simulink model "sixythree_level_modified"  (R2020a)
settings: Solver=ode45  StartTime=0.0  StopTime=0.02  RelTol=1e-3  EnableMultiTasking=on
libraries: powerlib x25
settings Model: Creator=harish  LastModifiedBy=sunil
settings DataIOCC: LimitDataPoints=on  SaveFormat=Array  ReturnWorkspaceOutputs=off
settings OptimizationCC: LifeSpan=inf
settings DebuggingCC: SFUnexpectedBacktrackingDiag=warning  SFNoUnconditionalDefaultTransitionDiag=warning  SFExecutionAtInitializationDiag=none  ArithmeticOperatorsInVariantConditions=warning
settings HardwareCC: ProdBitPerPointer=32  ProdBitPerSizeT=32  ProdBitPerPtrDiffT=32  ProdLargestAtomicFloat=None  ProdIntDivRoundTo=Undefined  ProdEndianess=Unspecified  ProdWordSize=32  ProdHWDeviceType=32-bit Generic
settings ModelReferenceCC: PropagateSignalLabelsOutOfModel=off
settings SFSimCC: SimUseLocalCustomCode=off  CustomCodeUndefinedFunction=UseInterfaceOnly
settings RTWCC: RTWUseLocalCustomCode=off
settings CodeAppCC: StateflowObjectComments=on
settings GRTTargetCC: TargetLangStandard=C89/C90 (ANSI)
settings ConfigComp: CovMetricSettings=dw  CovHtmlReporting=on  CovSaveCumulativeToWorkspaceVar=on  CovSaveSingleToWorkspaceVar=on  CovExternalEMLEnable=off
settings SimscapeCC: SimscapeNormalizeSystem=off

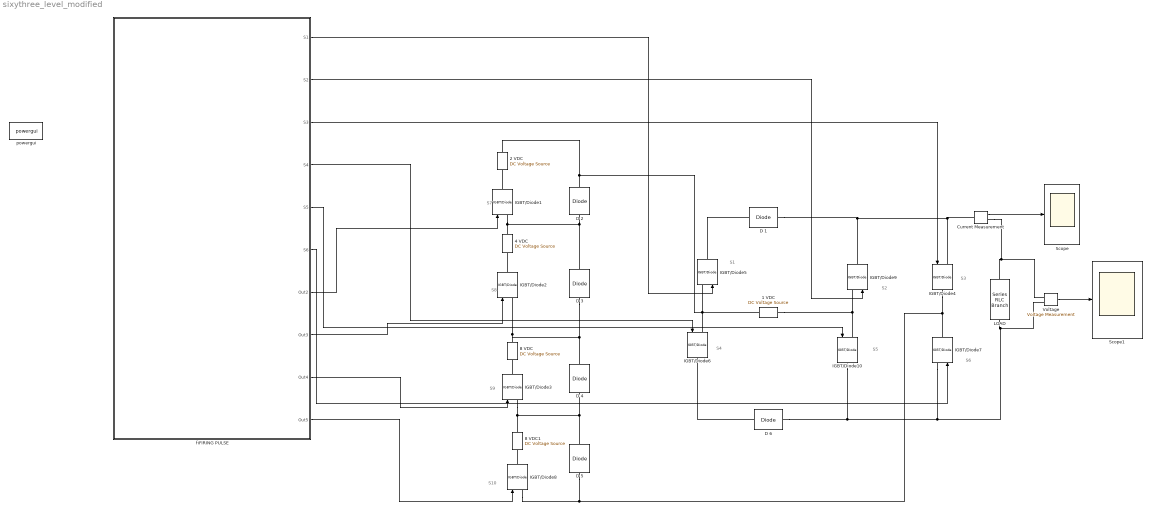
== system sixythree_level_modified ==
  note: S10
  note: S9
  note: S8
  note: S7
  note: S6
  note: S5
  note: S4
  note: S3
  note: S2
  note: S1
   D {1..6} (6 alike) : powerlib/Power Electronics/Diode  Ron=0.001  Lon=0  Vf=0.8  IC=0  UseSnubber=off  Rs=500  Cs=250e-9  Measurements=off
  "1 VDC " : powerlib/Electrical Sources/DC Voltage Source  Amplitude=240/31  Measurements=Voltage
  "2 VDC " : powerlib/Electrical Sources/DC Voltage Source  Amplitude=240*2/31  Measurements=Voltage
  "4 VDC " : powerlib/Electrical Sources/DC Voltage Source  Amplitude=240*4/31  Measurements=Voltage
  8 VDC : powerlib/Electrical Sources/DC Voltage Source  Amplitude=240*8/31  Measurements=Voltage
  8 VDC1 : powerlib/Electrical Sources/DC Voltage Source  Amplitude=240*16/31  Measurements=Voltage
  Current Measurement : powerlib/Measurements/Current Measurement  PhasorSimulation=off  OutputType=Complex  PSBequivalent=0
  IGBT/Diode{1..10} (10 alike) : powerlib/Power Electronics/IGBT//Diode  Ron=1e-3  Rs=1e5  Cs=inf  Measurements=off
  LOAD : powerlib/Elements/Series RLC Branch  LConnTagsString=__new0  RConnTagsString=__new0  BranchType=R  Resistance=100  Inductance=0.001  SetiL0=off  InitialCurrent=0  Capacitance=1e-6  Setx0=off  InitialVoltage=0  Measurements=None
  Scope : Scope
  Scope1 : Scope
  "Voltage " : powerlib/Measurements/Voltage Measurement  PhasorSimulation=off  OutputType=Complex  PSBequivalent=0
  fiFIRING PULSE : Subsystem
  powergui : powerlib/powergui  Priority=1  SimulationMode=Continuous  SampleTime=50e-6  frequency=60  Iterations=50  frequencyindice=0  Pbase=100e6  ErrMax=1e-4  UnitsV=kV  UnitsW=MW  buscounter=0  FunctionMessages=off  echomessages=off  EnableUseOfTLC=off  CurrentSourceSwitches=on  DisableSnubberDevices=off  DisableRonSwitches=off  DisableVfSwitches=off  DisplayEquations=off  AutomaticDiscreteSolvers=off  SolverType=Tustin/Backward Euler (TBE)  Interpol=off  ExternalGateDelay=off  methode=off  Ts=100  x0status=blocks  SPID=off  SwTol=0  HookPort=off  NonlinearTolerance=1e-4  nMaxIteration=100  ContinueOnMaxIteration=off  RestoreLinks=warning  ResistiveCurrentMeasurement=off  Frange=[0:2:500]  Ylog=off  Xlog=on  ShowGrid=off  save=off  variable=ZData  structure=voltage61  ZoomFFT=off  StartTime=0.0  cycles=1  DisplayStyle=1  fundamental=50  FreqAxis=on  MaxFrequency=1000  frequencyindicesteady=1  RmsSteady=1  display=off
  wires:
  "Voltage "/1 -> Scope1/1
  Current Measurement/1 -> Scope/1
  fiFIRING PULSE/10(Out5) -> IGBT/Diode8/1
  fiFIRING PULSE/9(Out4) -> IGBT/Diode3/1
  fiFIRING PULSE/8(Out3) -> IGBT/Diode2/1
  fiFIRING PULSE/7(Out2) -> IGBT/Diode1/1
  fiFIRING PULSE/1(S1) -> IGBT/Diode5/1
  fiFIRING PULSE/2(S2) -> IGBT/Diode9/1
  fiFIRING PULSE/3(S3) -> IGBT/Diode4/1
  fiFIRING PULSE/5(S5) -> IGBT/Diode10/1
  fiFIRING PULSE/6(S6) -> IGBT/Diode7/1
  fiFIRING PULSE/4(S4) -> IGBT/Diode6/1
  connections:
  " D 2"/LConn1 -- " D 3"/RConn1 -- "4 VDC "/RConn1 -- IGBT/Diode1/LConn1
  IGBT/Diode4/LConn1 -- " D 1"/RConn1 -- IGBT/Diode9/RConn1 -- Current Measurement/LConn1
  IGBT/Diode2/RConn1 -- "4 VDC "/LConn1
  IGBT/Diode1/RConn1 -- "2 VDC "/LConn1
  IGBT/Diode3/RConn1 -- 8 VDC/LConn1
  " D 4"/RConn1 -- IGBT/Diode2/LConn1 -- 8 VDC/RConn1 -- " D 3"/LConn1
  IGBT/Diode3/LConn1 -- 8 VDC1/RConn1 -- " D 4"/LConn1 -- " D 5"/RConn1
  LOAD/RConn1 -- Current Measurement/RConn1 -- "Voltage "/LConn1
  IGBT/Diode4/RConn1 -- " D 5"/LConn1 -- IGBT/Diode8/LConn1 -- IGBT/Diode7/RConn1
  IGBT/Diode8/RConn1 -- 8 VDC1/LConn1
  "Voltage "/LConn2 -- LOAD/LConn1 -- IGBT/Diode7/LConn1 -- IGBT/Diode10/RConn1 -- " D 6"/RConn1
  IGBT/Diode10/LConn1 -- IGBT/Diode9/LConn1 -- "1 VDC "/RConn1
  IGBT/Diode6/LConn1 -- "2 VDC "/RConn1 -- " D 2"/RConn1 -- "1 VDC "/LConn1 -- IGBT/Diode5/LConn1
  " D 1"/LConn1 -- IGBT/Diode5/RConn1
  " D 6"/LConn1 -- IGBT/Diode6/RConn1

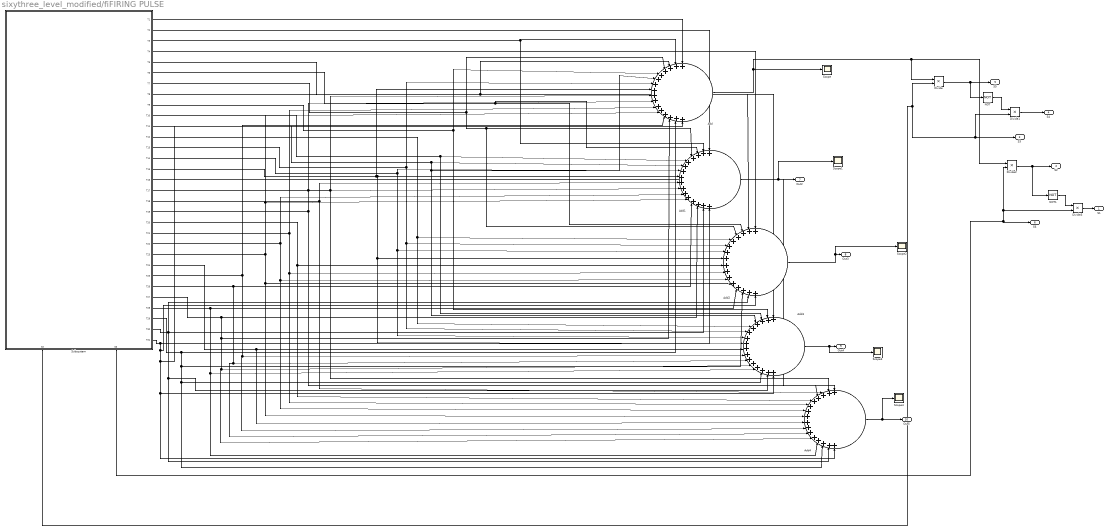
== system sixythree_level_modified/fiFIRING PULSE ==
  Add{,1..4} (5 alike) : Sum  Inputs=16
  Divide{,1..3} (4 alike) : Product  Inputs=**
  NOT : Logic  Operator=NOT  IconShape=distinctive  AllPortsSameDT=off  OutDataTypeStr=boolean
  NOT1 : Logic  Operator=NOT  IconShape=distinctive  AllPortsSameDT=off  OutDataTypeStr=boolean
  Scope{,1..4} (5 alike) : Scope
  Subsystem : Subsystem
      settings: PortSchema="{\"entries\":[{\"content\":{\"sides\":[{\"content\":{\"connectorIds\":[]},\"type\":\"ConnectorPlacement.EquallySpacedRectSide\",\"uuid\":\"70ad2b70-9561-48a4-a77f-34076edeb7a4\"},{\"content\":{\"connectorIds\":[\"Out1\",\"Out2\",\"Out3\",\"Out4\",\"Out5\",\"Out6\",\"Out7\",\"Out8\",\"Out9\",\"Out10\",\"Out11\",\"Out12\",\"Out13\",\"Out14\",\"Out15\",\"Out16\",\"Out17\",\"Out18\",\"Out19\",\"Out20\",\"Out21\",\"Out22\",\"Out23\",\"Out24\",\"Out25\",\"Out26\",\"Out27\",\"Out28\",\"Out29\",\"Out30\",\"Out31\"],\"side\":\"RIGHT\"},\"type\":\"ConnectorPlacement.EquallySpacedRectSide\",\"uuid\":\"b5d39657-1e04-4169-b553-b1962bf1f0e9\"},{\"content\":{\"connectorIds\":[],\"side\":\"TOP\"},\"type\":\"ConnectorPlacement.EquallySpacedRectSide\",\"uuid\":\"9b65afcb-07a6-4c10-8a50-7795185a824f\"},{\"content\":{\"connectorIds\":[\"Out32\",\"Out33\"],\"side\":\"BOTTOM\"},\"type\":\"ConnectorPlacement.EquallySpacedRectSide\",\"uuid\":\"1cd67243-db2c-4ba2-9ee1-558f28b37d25\"}]},\"type\":\"ConnectorPlacement.EquallySpacedConnector\",\"uuid\":\"3c7b11bc-dca1-47b6-888c-d1613d80d2b8\"}],\"packageUris\":[\"http://schema.mathworks.com/mf0/Connector/19700101\"],\"version\":\"1.0\"}"
  S1 : Outport
  S2 : Outport  Port=2
  S3 : Outport  Port=3
  S4 : Outport  Port=4
  S5 : Outport  Port=5
  S6 : Outport  Port=6
  Out2 : Outport  Port=7
  Out3 : Outport  Port=8
  Out4 : Outport  Port=9
  Out5 : Outport  Port=10
  wires:
  Subsystem/1(T1) -> Add/1
  Add/1 -> Scope/1, Divide2/1, Divide/1
  Add4/1 -> Scope4/1, Out5/1
  Add3/1 -> Scope3/1, Out4/1
  Add2/1 -> Scope2/1, Out3/1
  Add1/1 -> Out2/1, Scope1/1
  Subsystem/2(T2) -> Add1/1
  Subsystem/3(T3) -> Add1/2, Add/2
  Subsystem/4(T4) -> Add2/1
  Subsystem/5(T5) -> Add/3, Add2/2
  Subsystem/6(T6) -> Add1/3, Add2/3
  Subsystem/7(T7) -> Add/4, Add2/4, Add1/4
  Subsystem/8(T8) -> Add3/1
  Subsystem/9(T9) -> Add/5, Add3/2
  Subsystem/10(T10) -> Add3/3, Add1/5
  Subsystem/11(T11) -> Add/6, Add3/4, Add1/6
  Subsystem/12(T12) -> Add3/5, Add2/5
  Subsystem/13(T13) -> Add/7, Add3/6, Add2/6
  Subsystem/14(T14) -> Add3/7, Add2/7, Add1/7
  Subsystem/15(T15) -> Add3/8, Add2/8, Add1/8, Add/8
  Subsystem/16(T16) -> Add4/1
  Subsystem/17(T17) -> Add4/2, Add/9
  Subsystem/18(T18) -> Add4/3, Add1/9
  Subsystem/19(T19) -> Add4/4, Add1/10, Add/10
  Subsystem/20(T20) -> Add2/9, Add4/5
  Subsystem/21(T21) -> Add4/6, Add2/10, Add/11
  Subsystem/22(T22) -> Add2/11, Add4/7, Add1/11
  Subsystem/23(T23) -> Add4/8, Add2/12, Add/12, Add1/12
  Subsystem/24(T24) -> Add3/9, Add4/9
  Subsystem/32(" S3") -> Divide/2, Divide1/2, S3/1
  Subsystem/25(T25) -> Add4/10, Add3/10, Add/13
  Subsystem/26(T26) -> Add4/11, Add3/11, Add1/13
  Subsystem/27(T27) -> Add1/14, Add/14, Add4/12, Add3/12
  Subsystem/28(T28) -> Add4/13, Add3/13, Add2/13
  Subsystem/29(T29) -> Add/15, Add2/14, Add4/14, Add3/14
  Subsystem/30(T30) -> Add2/15, Add1/15, Add3/15, Add4/15
  Subsystem/31(T31) -> Add1/16, Add2/16, Add/16, Add4/16, Add3/16
  Subsystem/33(" S6") -> Divide2/2, Divide3/2, S6/1
  Divide/1 -> NOT/1, S5/1
  NOT/1 -> Divide1/1
  Divide1/1 -> S4/1
  NOT1/1 -> Divide3/1
  Divide2/1 -> NOT1/1, S2/1
  Divide3/1 -> S1/1

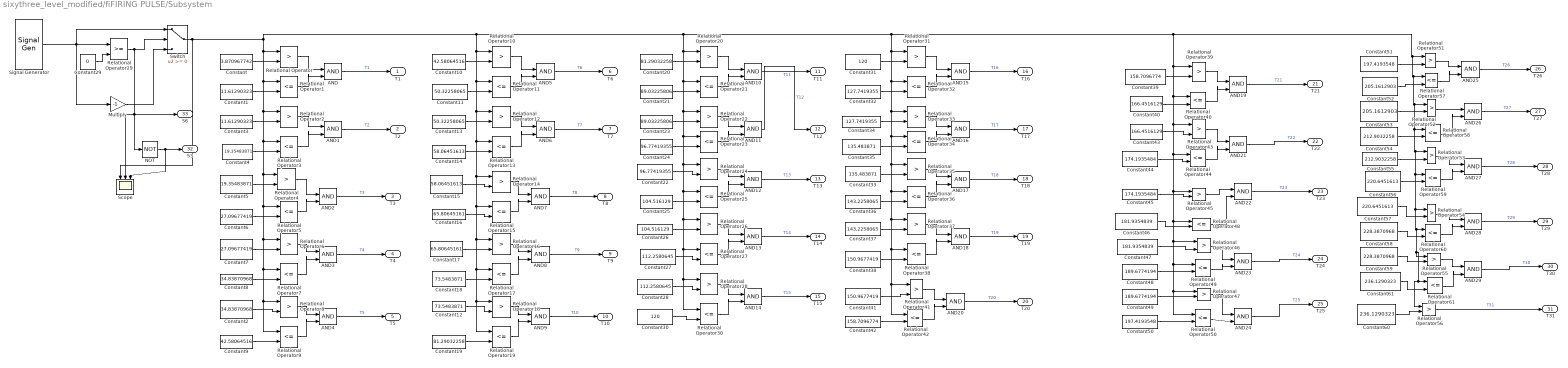
== system sixythree_level_modified/fiFIRING PULSE/Subsystem ==
  AND{,1..29} (30 alike) : Logic  IconShape=distinctive  AllPortsSameDT=off  OutDataTypeStr=boolean
  Constant : Constant  Value=3.870967742
  Constant1 : Constant  Value=11.61290323
  Constant10 : Constant  Value=42.58064516
  Constant11 : Constant  Value=50.32258065
  Constant12 : Constant  Value=73.5483871
  Constant13 : Constant  Value=50.32258065
  Constant14 : Constant  Value=58.06451613
  Constant15 : Constant  Value=58.06451613
  Constant16 : Constant  Value=65.80645161
  Constant17 : Constant  Value=65.80645161
  Constant18 : Constant  Value=73.5483871
  Constant19 : Constant  Value=81.29032258
  Constant2 : Constant  Value=34.83870968
  Constant20 : Constant  Value=81.29032258
  Constant21 : Constant  Value=89.03225806
  Constant22 : Constant  Value=96.77419355
  Constant23 : Constant  Value=89.03225806
  Constant24 : Constant  Value=96.77419355
  Constant25 : Constant  Value=104.516129
  Constant26 : Constant  Value=104.516129
  Constant27 : Constant  Value=112.2580645
  Constant28 : Constant  Value=112.2580645
  Constant29 : Constant  Value=0
  Constant3 : Constant  Value=11.61290323
  Constant30 : Constant  Value=120
  Constant31 : Constant  Value=120
  Constant32 : Constant  Value=127.7419355
  Constant33 : Constant  Value=135.483871
  Constant34 : Constant  Value=127.7419355
  Constant35 : Constant  Value=135.483871
  Constant36 : Constant  Value=143.2258065
  Constant37 : Constant  Value=143.2258065
  Constant38 : Constant  Value=150.9677419
  Constant39 : Constant  Value=158.7096774
  Constant4 : Constant  Value=19.35483871
  Constant40 : Constant  Value=166.4516129
  Constant41 : Constant  Value=150.9677419
  Constant42 : Constant  Value=158.7096774
  Constant43 : Constant  Value=166.4516129
  Constant44 : Constant  Value=174.1935484
  Constant45 : Constant  Value=174.1935484
  Constant46 : Constant  Value=181.9354839
  Constant47 : Constant  Value=181.9354839
  Constant48 : Constant  Value=189.6774194
  Constant49 : Constant  Value=189.6774194
  Constant5 : Constant  Value=19.35483871
  Constant50 : Constant  Value=197.4193548
  Constant51 : Constant  Value=197.4193548
  Constant52 : Constant  Value=205.1612903
  Constant53 : Constant  Value=205.1612903
  Constant54 : Constant  Value=212.9032258
  Constant55 : Constant  Value=212.9032258
  Constant56 : Constant  Value=220.6451613
  Constant57 : Constant  Value=220.6451613
  Constant58 : Constant  Value=228.3870968
  Constant59 : Constant  Value=228.3870968
  Constant6 : Constant  Value=27.09677419
  Constant60 : Constant  Value=236.1290323
  Constant61 : Constant  Value=236.1290323
  Constant7 : Constant  Value=27.09677419
  Constant8 : Constant  Value=34.83870968
  Constant9 : Constant  Value=42.58064516
  Multiply : Gain  Gain=-1
  NOT : Logic  Operator=NOT  IconShape=distinctive  AllPortsSameDT=off  OutDataTypeStr=boolean
  Relational Operator{,2,4,6,8,10,12,14,16,18,20,22,24,26,28,31,33,35,37,39,41,43,45..47,51..56} (31 alike) : RelationalOperator  Operator=>  OutDataTypeStr=boolean  RndMeth=Nearest
  Relational Operator{1,3,5,7,9,11,13,15,17,19,21,23,25,27,30,32,34,36,38,40,42,44,48..50,57..61} (30 alike) : RelationalOperator  Operator=<=  OutDataTypeStr=boolean  RndMeth=Nearest
  Relational Operator29 : RelationalOperator  OutDataTypeStr=boolean  RndMeth=Nearest
  Scope : Scope  NumInputPorts=3
  Signal Generator : SignalGenerator  Amplitude=240  Frequency=50
  Switch : Switch
  T1 : Outport
  T2 : Outport  Port=2
  T3 : Outport  Port=3
  T4 : Outport  Port=4
  T5 : Outport  Port=5
  T6 : Outport  Port=6
  T7 : Outport  Port=7
  T8 : Outport  Port=8
  T9 : Outport  Port=9
  T10 : Outport  Port=10
  T11 : Outport  Port=11
  T12 : Outport  Port=12
  T13 : Outport  Port=13
  T14 : Outport  Port=14
  T15 : Outport  Port=15
  T16 : Outport  Port=16
  T17 : Outport  Port=17
  T18 : Outport  Port=18
  T19 : Outport  Port=19
  T20 : Outport  Port=20
  T21 : Outport  Port=21
  T22 : Outport  Port=22
  T23 : Outport  Port=23
  T24 : Outport  Port=24
  T25 : Outport  Port=25
  T26 : Outport  Port=26
  T27 : Outport  Port=27
  T28 : Outport  Port=28
  T29 : Outport  Port=29
  T30 : Outport  Port=30
  T31 : Outport  Port=31
  " S3" : Outport  Port=32
  " S6" : Outport  Port=33
  wires:
  Relational Operator52/1 -> AND26/1
  Relational Operator7/1 -> AND3/2
  AND24/1 -> T25/1  "T25"
  Relational Operator55/1 -> AND29/1
  Signal Generator/1 -> Multiply/1, Switch/1, Relational Operator29/1
  AND19/1 -> T21/1  "T21"
  Constant21/1 -> Relational Operator21/2
  AND/1 -> T1/1  "T1"
  Constant36/1 -> Relational Operator36/2
  AND25/1 -> T26/1  "T26"
  Constant49/1 -> Relational Operator47/2
  Constant33/1 -> Relational Operator35/2
  Relational Operator29/1 -> Switch/2, " S6"/1, Scope/2, NOT/1
  Relational Operator31/1 -> AND15/1
  Constant13/1 -> Relational Operator12/2
  AND29/1 -> T30/1  "T30"
  AND8/1 -> T9/1  "T9"
  Relational Operator44/1 -> AND21/2
  Constant1/1 -> Relational Operator1/2
  AND28/1 -> T29/1  "T29"
  Constant/1 -> Relational Operator/2
  Constant58/1 -> Relational Operator60/2
  Constant10/1 -> Relational Operator10/2
  Constant19/1 -> Relational Operator19/2
  Constant48/1 -> Relational Operator49/2
  Constant57/1 -> Relational Operator54/2
  Relational Operator43/1 -> AND21/1
  Relational Operator54/1 -> AND28/1
  Relational Operator34/1 -> AND16/2
  Relational Operator16/1 -> AND8/1
  Relational Operator9/1 -> AND4/2
  AND23/1 -> T24/1  "T24"
  AND22/1 -> T23/1  "T23"
  Constant52/1 -> Relational Operator57/2
  Relational Operator5/1 -> AND2/2
  AND4/1 -> T5/1  "T5"
  AND26/1 -> T27/1  "T27"
  Constant25/1 -> Relational Operator25/2
  Relational Operator35/1 -> AND17/1
  Constant11/1 -> Relational Operator11/2
  Constant41/1 -> Relational Operator41/2
  Constant29/1 -> Relational Operator29/2
  Relational Operator23/1 -> AND11/2
  Relational Operator47/1 -> AND24/1
  Relational Operator37/1 -> AND18/1
  AND17/1 -> T18/1  "T18"
  Relational Operator60/1 -> AND28/2
  Constant43/1 -> Relational Operator43/2
  Relational Operator15/1 -> AND7/2
  Relational Operator59/1 -> AND27/2
  AND2/1 -> T3/1  "T3"
  Constant51/1 -> Relational Operator51/2
  Constant32/1 -> Relational Operator32/2
  AND11/1 -> T12/1  "T12"
  Constant9/1 -> Relational Operator9/2
  Relational Operator10/1 -> AND5/1
  Relational Operator49/1 -> AND23/2
  Constant27/1 -> Relational Operator27/2
  Constant38/1 -> Relational Operator38/2
  Constant31/1 -> Relational Operator31/2
  Relational Operator57/1 -> AND25/2
  Relational Operator51/1 -> AND25/1
  Constant53/1 -> Relational Operator52/2
  AND27/1 -> T28/1  "T28"
  AND6/1 -> T7/1  "T7"
  Relational Operator8/1 -> AND4/1
  Relational Operator45/1 -> AND22/1
  Constant55/1 -> Relational Operator53/2
  Relational Operator1/1 -> AND/2
  AND21/1 -> T22/1  "T22"
  Constant56/1 -> Relational Operator59/2
  Constant54/1 -> Relational Operator58/2
  Relational Operator11/1 -> AND5/2
  Relational Operator3/1 -> AND1/2
  Relational Operator26/1 -> AND13/1
  AND12/1 -> T13/1  "T13"
  Relational Operator20/1 -> AND10/1
  Relational Operator2/1 -> AND1/1
  Constant5/1 -> Relational Operator4/2
  Constant37/1 -> Relational Operator37/2
  Relational Operator22/1 -> AND11/1
  Constant20/1 -> Relational Operator20/2
  Constant40/1 -> Relational Operator40/2
  Constant26/1 -> Relational Operator26/2
  Relational Operator46/1 -> AND23/1
  Relational Operator39/1 -> AND19/1
  Relational Operator38/1 -> AND18/2
  Relational Operator50/1 -> AND24/2
  Constant22/1 -> Relational Operator24/2
  AND14/1 -> T15/1  "T15"
  Constant46/1 -> Relational Operator48/2
  Constant45/1 -> Relational Operator45/2
  Relational Operator41/1 -> AND20/1
  Constant39/1 -> Relational Operator39/2
  Multiply/1 -> Switch/3
  Relational Operator4/1 -> AND2/1
  Constant44/1 -> Relational Operator44/2
  Relational Operator48/1 -> AND22/2
  Relational Operator42/1 -> AND20/2
  Constant50/1 -> Relational Operator50/2
  Constant47/1 -> Relational Operator46/2
  Relational Operator24/1 -> AND12/1
  AND16/1 -> T17/1  "T17"
  Constant35/1 -> Relational Operator34/2
  AND10/1 -> T11/1  "T11"
  AND9/1 -> T10/1  "T10"
  Relational Operator21/1 -> AND10/2
  Constant42/1 -> Relational Operator42/2
  AND15/1 -> T16/1  "T16"
  Relational Operator40/1 -> AND19/2
  NOT/1 -> " S3"/1, Scope/3
  Relational Operator58/1 -> AND26/2
  Relational Operator12/1 -> AND6/1
  Constant16/1 -> Relational Operator15/2
  Relational Operator30/1 -> AND14/2
  Relational Operator32/1 -> AND15/2
  AND20/1 -> T20/1  "T20"
  Constant30/1 -> Relational Operator30/2
  AND18/1 -> T19/1  "T19"
  Constant28/1 -> Relational Operator28/2
  Relational Operator28/1 -> AND14/1
  Relational Operator27/1 -> AND13/2
  Constant15/1 -> Relational Operator14/2
  AND5/1 -> T6/1  "T6"
  Constant18/1 -> Relational Operator17/2
  Constant14/1 -> Relational Operator13/2
  AND1/1 -> T2/1  "T2"
  Constant6/1 -> Relational Operator5/2
  AND13/1 -> T14/1  "T14"
  Constant34/1 -> Relational Operator33/2
  Relational Operator14/1 -> AND7/1
  Relational Operator17/1 -> AND8/2
  Constant2/1 -> Relational Operator8/2
  Relational Operator33/1 -> AND16/1
  Relational Operator19/1 -> AND9/2
  Relational Operator6/1 -> AND3/1
  AND7/1 -> T8/1  "T8"
  Constant17/1 -> Relational Operator16/2
  Relational Operator18/1 -> AND9/1
  Constant24/1 -> Relational Operator23/2
  Relational Operator36/1 -> AND17/2
  Constant23/1 -> Relational Operator22/2
  Relational Operator13/1 -> AND6/2
  Relational Operator53/1 -> AND27/1
  Constant8/1 -> Relational Operator7/2
  Relational Operator/1 -> AND/1
  Constant3/1 -> Relational Operator2/2
  AND3/1 -> T4/1  "T4"
  Relational Operator25/1 -> AND12/2
  Constant12/1 -> Relational Operator18/2
  Constant4/1 -> Relational Operator3/2
  Constant7/1 -> Relational Operator6/2
  Constant59/1 -> Relational Operator55/2
  Switch/1 -> Relational Operator39/1, Relational Operator43/1, Relational Operator45/1, Relational Operator48/1, Relational Operator46/1, Relational Operator49/1, Relational Operator47/1, Relational Operator50/1, Relational Operator44/1, Relational Operator40/1, Relational Operator58/1, Relational Operator56/1, Relational Operator61/1, Relational Operator55/1, Relational Operator60/1, Relational Operator54/1, Relational Operator59/1, Relational Operator53/1, Relational Operator52/1, Relational Operator57/1, Relational Operator51/1, Relational Operator31/1, Relational Operator33/1, Relational Operator35/1, Relational Operator37/1, Relational Operator38/1, Relational Operator41/1, Relational Operator42/1, Relational Operator36/1, Relational Operator34/1, Relational Operator32/1, Relational Operator20/1, Relational Operator22/1, Relational Operator24/1, Relational Operator26/1, Relational Operator28/1, Relational Operator30/1, Relational Operator27/1, Relational Operator25/1, Relational Operator23/1, Relational Operator21/1, Relational Operator10/1, Relational Operator12/1, Relational Operator18/1, Relational Operator19/1, Relational Operator17/1, Relational Operator16/1, Relational Operator15/1, Relational Operator14/1, Relational Operator13/1, Relational Operator11/1, Relational Operator/1, Relational Operator2/1, Relational Operator8/1, Relational Operator9/1, Relational Operator7/1, Relational Operator6/1, Relational Operator5/1, Relational Operator4/1, Relational Operator3/1, Relational Operator1/1, Scope/1
  Relational Operator56/1 -> T31/1  "T31"
  Constant60/1 -> Relational Operator56/2
  Constant61/1 -> Relational Operator61/2
  Relational Operator61/1 -> AND29/2
